simulink model "franka_Simulink_ROS_Control"  (R2022b)
settings: Solver=FixedStepAuto  StartTime=0.0  StopTime=25  FixedStep=0.1  RelTol=1e-3
PreLoadFcn:
  | %robot = importrobot("panda_model.urdf"); %create rigid body tree object shared on ROS from /tf
model workspace (MAT data in the model file):
  SL_ROS_VariableLengthArrays_MaxSizes.CommonInfo.ArrayTruncateAction = 'EmitWarning'
  SL_ROS_VariableLengthArrays_MaxSizes.MsgTypeMap = containers.Map
  SL_ROS_VariableLengthArrays_MaxSizes.MsgTypeMap.serialization.keys = {'sensor_msgs/Image'}
  SL_ROS_VariableLengthArrays_MaxSizes.MsgTypeMap.serialization.values{1}(1).PropertyName = 'Data'
  SL_ROS_VariableLengthArrays_MaxSizes.MsgTypeMap.serialization.values{1}(1).DataType = 'uint8'
  SL_ROS_VariableLengthArrays_MaxSizes.MsgTypeMap.serialization.values{1}(1).MaxLength = 1228800
  SL_ROS_VariableLengthArrays_MaxSizes.MsgTypeMap.serialization.values{1}(2).PropertyName = 'Encoding'
  SL_ROS_VariableLengthArrays_MaxSizes.MsgTypeMap.serialization.values{1}(2).DataType = 'uint8'
  SL_ROS_VariableLengthArrays_MaxSizes.MsgTypeMap.serialization.values{1}(2).MaxLength = 128
  SL_ROS_VariableLengthArrays_MaxSizes.MsgTypeMap.serialization.uniformity = 0
  SL_ROS_VariableLengthArrays_MaxSizes.MsgTypeMap.serialization.keyType = 'char'
  SL_ROS_VariableLengthArrays_MaxSizes.MsgTypeMap.serialization.valueType = 'any'
undefined symbols (not defined in the file or in its folder): gray
libraries: robotlib x6, robotgazebolib x1
settings Model: Creator=amavromm  LastModifiedBy=josea
settings SolverCC: AlgebraicLoopSolver=TrustRegion
settings OptimizationCC: EnhancedBackFolding=on  PassReuseOutputArgsAs=Individual arguments  ZeroExternalMemoryAtStartup=off  ZeroInternalMemoryAtStartup=off  MaxStackSize=64  OptimizeBlockOrder=speed  DifferentSizesBufferReuse=on  OptimizationCustomize=off  EfficientTunableParamExpr=on
settings DebuggingCC: ParameterTunabilityLossMsg=error  UnconnectedInputMsg=warning  UnconnectedOutputMsg=warning  UnconnectedLineMsg=warning  SFMachineParentedDataDiag=warning
settings HardwareCC: ProdBitPerPointer=32  ProdBitPerSizeT=32  ProdBitPerPtrDiffT=32  ProdLargestAtomicFloat=None  ProdIntDivRoundTo=Undefined  ProdEndianess=Unspecified  ProdWordSize=32  ProdHWDeviceType=Generic->Unspecified (assume 32-bit Generic)
settings ModelReferenceCC: EnableRefExpFcnMdlSchedulingChecks=on
settings SFSimCC: MATLABDynamicMemAlloc=off  SimTargetLang=C++
settings RTWCC: Description=Embedded Coder  SystemTargetFile=ert.tlc  HardwareBoard=Robot Operating System (ROS)  TLCOptions="-aInlineSetEventsForThisBaseRateFcn=TLC_FALSE -aSuppressMultiTaskScheduler=TLC_FALSE  -aRateBasedStepFcn=0"  TemplateMakefile=ert_default_tmf  Toolchain=Catkin  TargetLang=C++  DLArmComputeVersion=19.05
settings CodeAppCC: ForceParamTrailComments=on  IgnoreCustomStorageClasses=off  OperatorAnnotations=on  SimulinkDataObjDesc=on  SFDataObjDesc=on  InsertBlockDesc=on

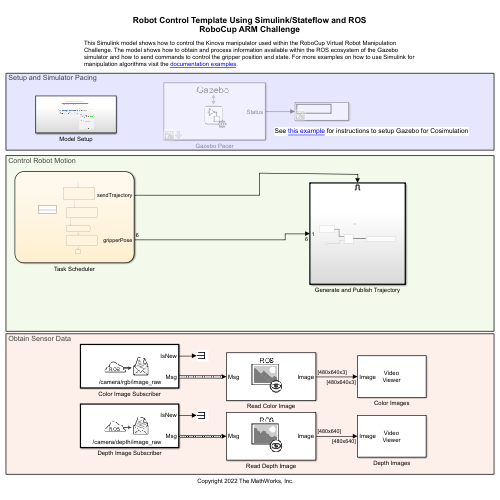
[thumbnail: Simulink's stored preview of the top-level diagram]
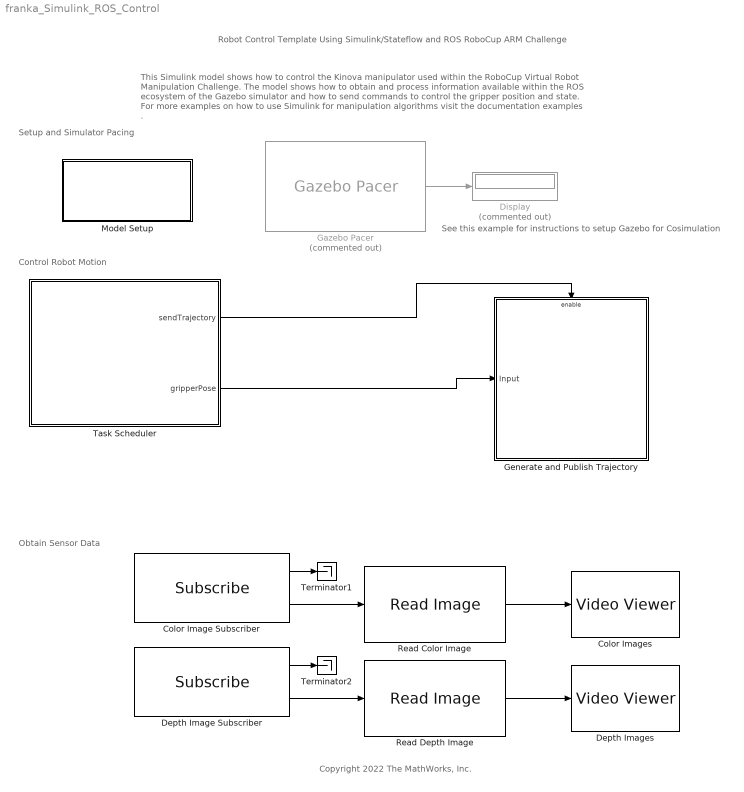
== system franka_Simulink_ROS_Control ==
  note: See this example for instructions to setup Gazebo for Cosimulation
  note: This Simulink model shows how to control the Kinova manipulator used within the RoboCup Virtual Robot Manipulation Challenge. The model shows how to obtain and process information available within the ROS ecosystem of the Gazebo simulator and how to send commands to control the gripper position and state. For more examples on how to use Simulink for manipulation algorithms visit the documentation examples .
  note: Robot Control Template Using Simulink/Stateflow and ROS
      | RoboCup ARM Challenge
  note: Obtain Sensor Data
  note: Control Robot Motion
  note: Setup and Simulator Pacing
  note: Copyright 2022 The MathWorks, Inc.
  Color Image Subscriber : robotlib/Subscribe  topicSource=Select from ROS network  topic=/camera/rgb/image_raw  messageType=sensor_msgs/Image  SampleTime=0.5  legacyBusStruct=off  messageQueueLength=1
  Color Images : VideoViewer  colormapValue=gray(256)  FigPos=[1482 504 418 304]
  Depth Image Subscriber : robotlib/Subscribe  topicSource=Select from ROS network  topic=/camera/depth/image_raw  messageType=sensor_msgs/Image  SampleTime=0.5  legacyBusStruct=off  messageQueueLength=1
  Depth Images : VideoViewer  colormapValue=gray(256)  FigPos=[1427 943 418 304]
  Display : Display  Commented=on
  Gazebo Pacer : robotgazebolib/Gazebo Pacer  Commented=on  ResetBehavior=Reset Gazebo simulation time  SampleTime=0.1
  Generate and Publish Trajectory : Subsystem
  Model Setup : Subsystem
  Read Color Image : robotlib/Read Image  MaximumImageSize=[480, 640]  ImageEncoding=rgb8  ShowAlphaOutput=off  ShowErrorCodeOutput=off  VariableSizeOutputs=off
  Read Depth Image : robotlib/Read Image  MaximumImageSize=[480, 640]  ImageEncoding=32fc1  ShowAlphaOutput=off  ShowErrorCodeOutput=off  VariableSizeOutputs=off
  Task Scheduler : Stateflow chart  TreatAsAtomicUnit=on
  Terminator1 : Terminator
  Terminator2 : Terminator
  wires:
  Task Scheduler/1(sendTrajectory) -> Generate and Publish Trajectory/Enable
  Task Scheduler/2(gripperPose) -> Generate and Publish Trajectory/1(Input)
  Gazebo Pacer/1 -> Display/1
  Color Image Subscriber/2 -> Read Color Image/1
  Color Image Subscriber/1 -> Terminator1/1
  Read Color Image/1 -> Color Images/1
  Depth Image Subscriber/2 -> Read Depth Image/1
  Read Depth Image/1 -> Depth Images/1
  Depth Image Subscriber/1 -> Terminator2/1

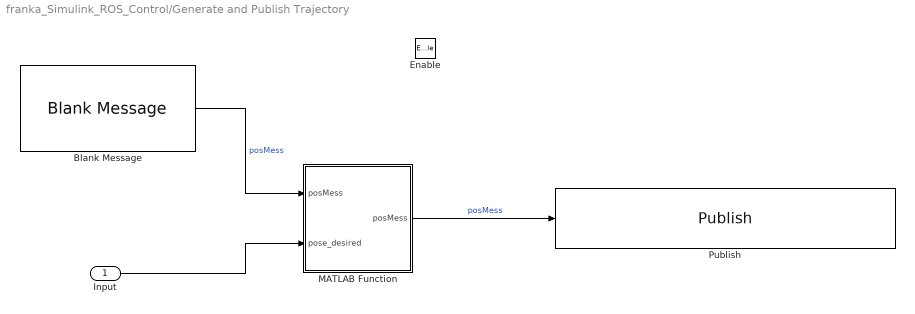
== system franka_Simulink_ROS_Control/Generate and Publish Trajectory ==
  Input : Inport
  Enable : EnablePort
  Blank Message : robotlib/Blank Message  messageClass=Message  entityType=geometry_msgs/PoseStamped  messageType=geometry_msgs/PoseStamped  SampleTime=inf  legacyBusStruct=off
  MATLAB Function : MATLAB Function  TreatAsAtomicUnit=on
  Publish : robotlib/Publish  topicSource=Select from ROS network  topic=/cartesian_impedance_example_controller/equilibrium_pose  messageType=geometry_msgs/PoseStamped  legacyBusStruct=off  messageQueueLength=1
  wires:
  Blank Message/1 -> MATLAB Function/1("posMess ")  "posMess"
  Input/1 -> MATLAB Function/2(pose_desired)
  MATLAB Function/1(posMess) -> Publish/1  "posMess"

== system franka_Simulink_ROS_Control/Model Setup ==
  note: 1
  note: Before running the Simulink model, make sure the ROS network requirements have been set appropriately through the Simulink Toolstrip and MATLAB ROS Node has been initiated. Note that setting a Node Host IP address is optional and depends on the computer setup.
  note: ROS Model Setup
  note: 22
  note: 23

== matlab function franka_Simulink_ROS_Control/Generate and Publish Trajectory/MATLAB Function ==
  data: posMess input Bus: SL_Bus_franka_Simulink_ROS_Contr_PoseStamped_e9as7u; posMess output; pose_desired input
function posMess = packageTrajectory(posMess,pose_desired)

coder.extrinsic('angle2quat');
posMess.Pose.Position.X = pose_desired(1);
posMess.Pose.Position.Y =  pose_desired(2);
posMess.Pose.Position.Z =  pose_desired(3);
quat = angle2quat( pose_desired(4),  pose_desired(5),  pose_desired(6), "XYZ");
posMess.Pose.Orientation.W = quat(1);
posMess.Pose.Orientation.X = quat(2);
posMess.Pose.Orientation.Y = quat(3);
posMess.Pose.Orientation.Z = quat(4);

end

== stateflow chart franka_Simulink_ROS_Control/Task Scheduler ==
  state Initialize
    gripperPose = [0.4 0 0.4 -pi -0.01 0]';
    sendTrajectory = 0;
    activateGripper(1);
  state MoveForward
    entry:
    gripperPose = [0.7 0 0.4 -pi -0.01 0]';
    during:
    sendTrajectory =1;
  state CloseGripper
    activateGripper(0);
  state MoveBackward
    entry:
    gripperPose = [0.4 0 0.4 -pi -0.01 0]';
    during:
    sendTrajectory = 1;
  state Idle
  (default) -> Initialize : {activateGripper(2);}
      | % Initialize Gripper Action Client
  Initialize -> MoveForward : [after(5,sec)]
  MoveForward -> CloseGripper : [after(4,sec)] {sendTrajectory=0;}
      | % Wait for trajectory following controller and disable
  CloseGripper -> MoveBackward : [after(4,sec)]
  MoveBackward -> Idle : [after(4,sec)] {sendTrajectory=0;}
  data: state function_input; sendTrajectory output; gripperPose output
  function activateGripper(state):
    | function activateGripper(state)
    |   coder.extrinsic('frankaSLActivateGripper')
    |   frankaSLActivateGripper(state)
    | end
